simulink model "g_vector"  (R2016b)
settings: Solver=ode45  StartTime=0.0  StopTime=10.0  RelTol=1e-3  EnableMultiTasking=on
values from neighbouring files (symbols this model uses):
  a_1 = 1    [parameters.m]
  gravity = 9.81    [parameters.m]
  l_1 = 0.5    [parameters.m]
  l_2 = 0.5    [parameters.m]
  m_l_1 = 50    [parameters.m]
  m_l_2 = 50    [parameters.m]
  m_m_2 = 5    [parameters.m]
settings Model: Creator=kma  LastModifiedBy=kma
settings DataIOCC: LimitDataPoints=on  SaveFormat=Array
settings OptimizationCC: LifeSpan=inf
settings DebuggingCC: SFUnexpectedBacktrackingDiag=warning  SFNoUnconditionalDefaultTransitionDiag=warning  SFExecutionAtInitializationDiag=none
settings HardwareCC: ProdBitPerPointer=32  ProdBitPerSizeT=32  ProdBitPerPtrDiffT=32  ProdLargestAtomicFloat=None  ProdIntDivRoundTo=Undefined  ProdEndianess=Unspecified  ProdWordSize=32  ProdHWDeviceType=32-bit Generic
settings ModelReferenceCC: PropagateSignalLabelsOutOfModel=off
settings GRTTargetCC: TargetLangStandard=C89/C90 (ANSI)  GeneratePreprocessorConditionals=Disable all
settings ConfigComp: CovMetricSettings=dw  CovHtmlReporting=on  CovSaveCumulativeToWorkspaceVar=on  CovSaveSingleToWorkspaceVar=on  CovExternalEMLEnable=off

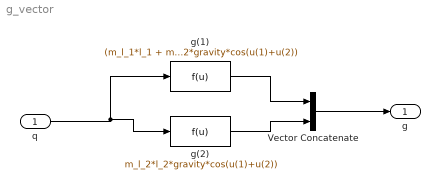
== system g_vector ==
  q : Inport  PortDimensions=2
  Vector Concatenate : Concatenate
  g(1) : Fcn  Expr=(m_l_1*l_1 + m_m_2*a_1 + m_l_2*a_1)*gravity*cos(u(1)) + m_l_2*l_2*gravity*cos(u(1)+u(2))
  g(2) : Fcn  Expr=m_l_2*l_2*gravity*cos(u(1)+u(2))
  g : Outport  PortDimensions=2
  wires:
  q/1 -> g(2)/1, g(1)/1
  Vector Concatenate/1 -> g/1
  g(2)/1 -> Vector Concatenate/2
  g(1)/1 -> Vector Concatenate/1
